simulink library "TestLib_BCM_Manager"  (Simulink 7.5)
settings: Solver=ode1  StartTime=0.0  StopTime=Inf  FixedStep=0.001  RelTol=1e-3
PostLoadFcn:
  | , if any(exist('dsrtsu_mdlpostloadfcn', 'file') == [2, 3, 6]), try dsrtsu_mdlpostloadfcn('Execute', bdroot); catch fprintf('Error in PostLoadFcn (dsrtsu_mdlpostloadfcn) for model "%s":\n %s\n', bdroot, lasterr); end, end,
undefined symbols (not defined in the file): cal, tloop
libraries: simulink x92, EC2_libraries x74
(part 1 of 2)
settings Model: DSRTSU_INTERNAL_RTI_VER=380  DSRTSU_INTERNAL_RTI_TYPE=rti1006  RTICANMMDATA=struct('GeneralSetupData',struct('modelroot',['C:\Users\EC2user\Documents\SVN__Controls\ecocar2_Controls\PTTR Alpha Branch\Libraries\CAN'],'generalsettings',struct('filesettings',struct('destfolder',struct('Name','RTICANMM_FILES','Check',1),'buildfolder',struct('Name','.','Check',1),'AbsDestfolder',struct('Name',['C:\Users\EC2user\Documents\SVN__Controls\ecocar2_Controls\PTTR Alpha Branch\Libraries\Diagnostics\Testing\RTICANMM_FILES']),'AbsBuildfolder',struct('Name',['C:\Users\EC2user\Documents\SVN__Controls\ecocar2_Controls\PTTR Alpha Branch\Libraries\CAN']))),'options',struct('addpaths',1,'rmpaths',1,'addtrcexclusion',logical(1),'cannavigator',struct('checkmonitoring',0,'serviceno','31','hostservicedefheader',struct('name','x','path','x')),'show_usrtrc',0,'use_usrtrc',0),'advanced',struct('options',[1 1 1 1 1 1 1 1 1 1 1 1 1 1 1 1 1 1 1 1 1 1 1 1 1 1 1 1 1 1 1 1 1 1 1 1 1 1 1 1 1 1 1 1 1 1 1 1 1 1 1 1 1 1 1 1 1 1 1 1 1 1 1 1 1 1 1 1 1 1 1 1 1 1 1 1 1 1 1 1 1 1 1 1 1 1 1 1 1 1 1 1 1 1 1 1 1 1 1 1]),'MPSetup',{{}},'modelname','DIAG_CAN_OUT','block','TestLib_BCM_Manager'))  Creator=idan  LastModifiedBy=Yuxia^_^

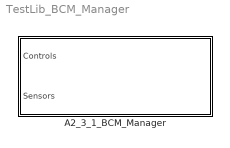
== system TestLib_BCM_Manager ==
  A2_3_1_BCM_Manager : Subsystem

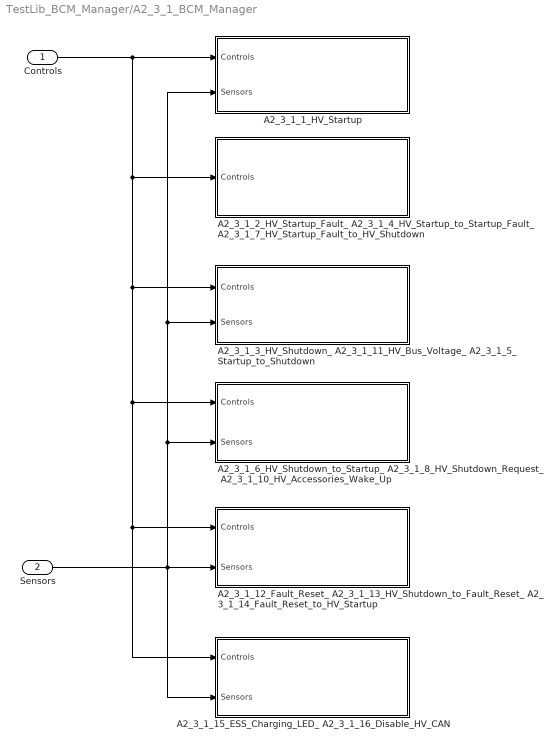
== system TestLib_BCM_Manager/A2_3_1_BCM_Manager ==
  Controls : Inport  OutDataType=fixdt(1, 16)  OutScaling=2^0
  Sensors : Inport  Port=2  OutDataType=fixdt(1, 16)  OutScaling=2^0
  A2_3_1_12_Fault_Reset_ A2_3_1_13_HV_Shutdown_to_Fault_Reset_ A2_3_1_14_Fault_Reset_to_HV_Startup : Subsystem
  A2_3_1_15_ESS_Charging_LED_ A2_3_1_16_Disable_HV_CAN : Subsystem
  A2_3_1_1_HV_Startup : Subsystem
  A2_3_1_2_HV_Startup_Fault_ A2_3_1_4_HV_Startup_to_Startup_Fault_ A2_3_1_7_HV_Startup_Fault_to_HV_Shutdown : Subsystem
  A2_3_1_3_HV_Shutdown_ A2_3_1_11_HV_Bus_Voltage_ A2_3_1_5_Startup_to_Shutdown : Subsystem
  A2_3_1_6_HV_Shutdown_to_Startup_ A2_3_1_8_HV_Shutdown_Request_ A2_3_1_10_HV_Accessories_Wake_Up : Subsystem
  wires:
  Controls/1 -> A2_3_1_15_ESS_Charging_LED_ A2_3_1_16_Disable_HV_CAN/1(Controls), A2_3_1_12_Fault_Reset_ A2_3_1_13_HV_Shutdown_to_Fault_Reset_ A2_3_1_14_Fault_Reset_to_HV_Startup/1(Controls), A2_3_1_6_HV_Shutdown_to_Startup_ A2_3_1_8_HV_Shutdown_Request_ A2_3_1_10_HV_Accessories_Wake_Up/1(Controls), A2_3_1_3_HV_Shutdown_ A2_3_1_11_HV_Bus_Voltage_ A2_3_1_5_Startup_to_Shutdown/1(Controls), A2_3_1_2_HV_Startup_Fault_ A2_3_1_4_HV_Startup_to_Startup_Fault_ A2_3_1_7_HV_Startup_Fault_to_HV_Shutdown/1(Controls), A2_3_1_1_HV_Startup/1(Controls)
  Sensors/1 -> A2_3_1_15_ESS_Charging_LED_ A2_3_1_16_Disable_HV_CAN/2(Sensors), A2_3_1_12_Fault_Reset_ A2_3_1_13_HV_Shutdown_to_Fault_Reset_ A2_3_1_14_Fault_Reset_to_HV_Startup/2(Sensors), A2_3_1_6_HV_Shutdown_to_Startup_ A2_3_1_8_HV_Shutdown_Request_ A2_3_1_10_HV_Accessories_Wake_Up/2(Sensors), A2_3_1_3_HV_Shutdown_ A2_3_1_11_HV_Bus_Voltage_ A2_3_1_5_Startup_to_Shutdown/2(Sensors), A2_3_1_1_HV_Startup/2(Sensors)

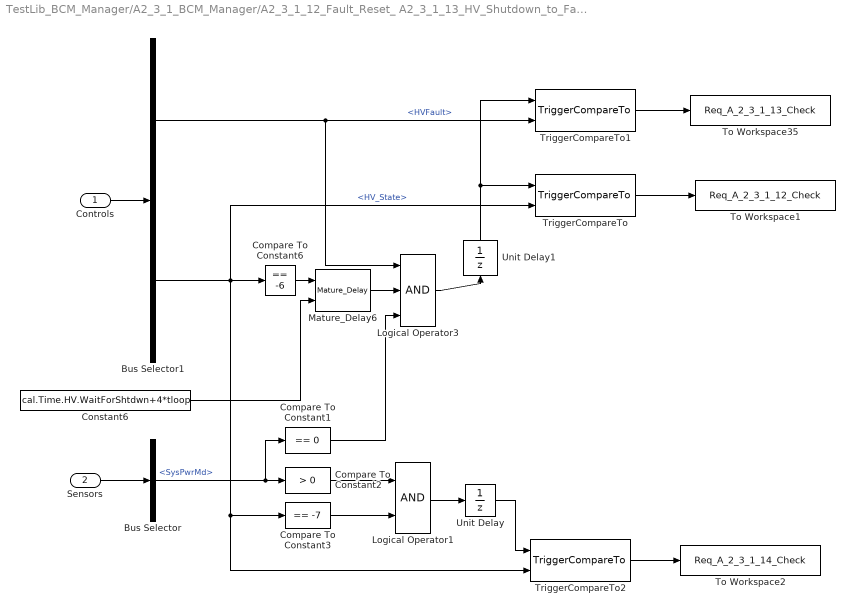
== system TestLib_BCM_Manager/A2_3_1_BCM_Manager/A2_3_1_12_Fault_Reset_ A2_3_1_13_HV_Shutdown_to_Fault_Reset_ A2_3_1_14_Fault_Reset_to_HV_Startup ==
  Controls : Inport  OutDataType=fixdt(1, 16)  OutScaling=2^0
  Sensors : Inport  Port=2  OutDataType=fixdt(1, 16)  OutScaling=2^0
  Bus Selector : BusSelector  OutputSignals=Sensors_CAN.BodyCM_HS_Tx.PPEI_Platform_General_Status.SysPwrMd
  Bus Selector1 : BusSelector  OutputSignals=Powertrain_SC_Controls.HV_Status.HVFault,Powertrain_SC_Controls.HV_Status.HV_State
  Compare To Constant1 : simulink/Logic and Bit Operations/Compare To Constant  SystemSampleTime=-1  relop===  const=0  LogicOutDataTypeMode=uint8
  Compare To Constant2 : simulink/Logic and Bit Operations/Compare To Constant  SystemSampleTime=-1  relop=>  const=0  LogicOutDataTypeMode=uint8
  Compare To Constant3 : simulink/Logic and Bit Operations/Compare To Constant  SystemSampleTime=-1  relop===  const=-7  LogicOutDataTypeMode=uint8
  Compare To Constant6 : simulink/Logic and Bit Operations/Compare To Constant  SystemSampleTime=-1  relop===  const=-6  LogicOutDataTypeMode=uint8
  Constant6 : Constant  Value=cal.Time.HV.WaitForShtdwn+4*tloop  VectorParams1D=off
  Logical Operator1 : Logic  AllPortsSameDT=off  OutDataTypeMode=boolean  OutDataTypeStr=boolean
  Logical Operator3 : Logic  Inputs=3  AllPortsSameDT=off  OutDataTypeMode=boolean  OutDataTypeStr=boolean
  Mature_Delay6 : EC2_libraries/Mature_Delay  SystemSampleTime=-1
  To Workspace1 : ToWorkspace  VariableName=Req_A_2_3_1_12_Check  SampleTime=-1  SaveFormat=Array
      settings: Decimation=WORKSPACE_DECIMATION
  To Workspace2 : ToWorkspace  VariableName=Req_A_2_3_1_14_Check  SampleTime=-1  SaveFormat=Array
      settings: Decimation=WORKSPACE_DECIMATION
  To Workspace35 : ToWorkspace  VariableName=Req_A_2_3_1_13_Check  SampleTime=-1  SaveFormat=Array
      settings: Decimation=WORKSPACE_DECIMATION
  TriggerCompareTo : EC2_libraries/TriggerCompareTo  SystemSampleTime=-1  exp_val=-7
  TriggerCompareTo1 : EC2_libraries/TriggerCompareTo  SystemSampleTime=-1  exp_val=0
  TriggerCompareTo2 : EC2_libraries/TriggerCompareTo  SystemSampleTime=-1  exp_val=-7
  Unit Delay : UnitDelay  SampleTime=-1
  Unit Delay1 : UnitDelay  SampleTime=-1
  wires:
  Unit Delay/1 -> TriggerCompareTo2/1
  Logical Operator1/1 -> Unit Delay/1
  Compare To Constant3/1 -> Logical Operator1/2
  Compare To Constant2/1 -> Logical Operator1/1
  TriggerCompareTo2/1 -> To Workspace2/1
  Logical Operator3/1 -> Unit Delay1/1
  TriggerCompareTo1/1 -> To Workspace35/1
  Bus Selector/1 -> Compare To Constant2/1, Compare To Constant1/1  "<SysPwrMd>"
  Bus Selector1/2 -> TriggerCompareTo/2, TriggerCompareTo2/2, Compare To Constant3/1, Compare To Constant6/1  "<HV_State>"
  Bus Selector1/1 -> TriggerCompareTo1/2, Logical Operator3/1  "<HVFault>"
  Controls/1 -> Bus Selector1/1
  Sensors/1 -> Bus Selector/1
  TriggerCompareTo/1 -> To Workspace1/1
  Unit Delay1/1 -> TriggerCompareTo1/1, TriggerCompareTo/1
  Compare To Constant1/1 -> Logical Operator3/3
  Constant6/1 -> Mature_Delay6/2
  Compare To Constant6/1 -> Mature_Delay6/1
  Mature_Delay6/1 -> Logical Operator3/2

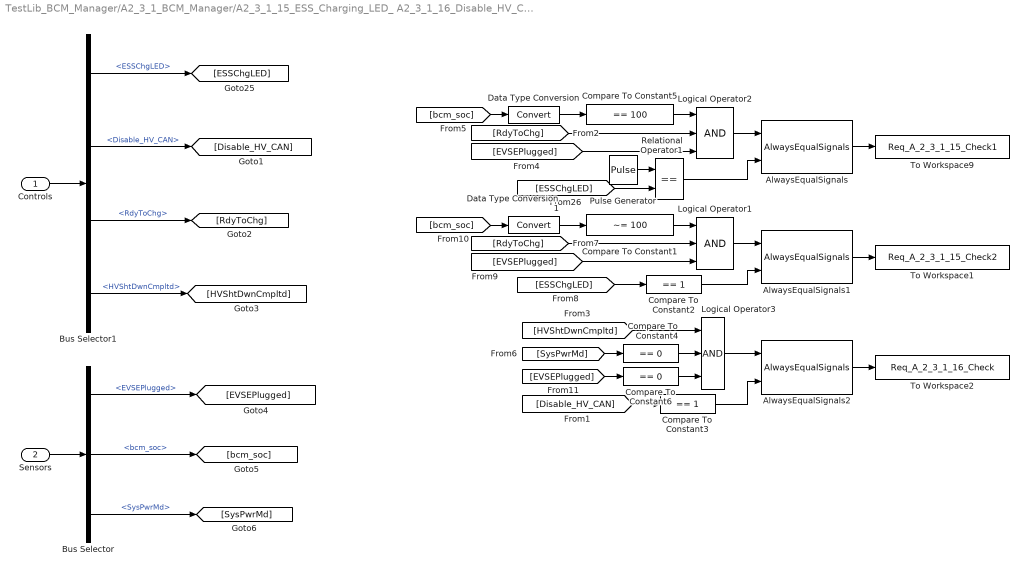
== system TestLib_BCM_Manager/A2_3_1_BCM_Manager/A2_3_1_15_ESS_Charging_LED_ A2_3_1_16_Disable_HV_CAN ==
  Controls : Inport  OutDataType=fixdt(1, 16)  OutScaling=2^0
  Sensors : Inport  Port=2  OutDataType=fixdt(1, 16)  OutScaling=2^0
  AlwaysEqualSignals : EC2_libraries/AlwaysEqualSignals  SystemSampleTime=-1
  AlwaysEqualSignals1 : EC2_libraries/AlwaysEqualSignals  SystemSampleTime=-1
  AlwaysEqualSignals2 : EC2_libraries/AlwaysEqualSignals  SystemSampleTime=-1
  Bus Selector : BusSelector  OutputSignals=Analog.EVSEPlugged,Sensors_CAN.BCM_HS_Tx.BCM_Status.bcm_soc,Sensors_CAN.BodyCM_HS_Tx.PPEI_Platform_General_Status.SysPwrMd
  Bus Selector1 : BusSelector  OutputSignals=Powertrain_SC_Controls.BCM_Control.ESSChgLED,Powertrain_SC_Controls.BCM_Control.Disable_HV_CAN,Powertrain_SC_Controls.HV_Status.RdyToChg,Powertrain_SC_Controls.HV_Status.HVShtDwnCmpltd
  Compare To Constant1 : simulink/Logic and Bit Operations/Compare To Constant  SystemSampleTime=-1  relop=~=  const=100  LogicOutDataTypeMode=boolean
  Compare To Constant2 : simulink/Logic and Bit Operations/Compare To Constant  SystemSampleTime=-1  relop===  const=1  LogicOutDataTypeMode=boolean
  Compare To Constant3 : simulink/Logic and Bit Operations/Compare To Constant  SystemSampleTime=-1  relop===  const=1  LogicOutDataTypeMode=boolean
  Compare To Constant4 : simulink/Logic and Bit Operations/Compare To Constant  SystemSampleTime=-1  relop===  const=0  LogicOutDataTypeMode=boolean
  Compare To Constant5 : simulink/Logic and Bit Operations/Compare To Constant  SystemSampleTime=-1  relop===  const=100  LogicOutDataTypeMode=boolean
  Compare To Constant6 : simulink/Logic and Bit Operations/Compare To Constant  SystemSampleTime=-1  relop===  const=0  LogicOutDataTypeMode=boolean
  Data Type Conversion : DataTypeConversion  OutDataType=fixdt(1, 16)  OutScaling=2^0
  Data Type Conversion1 : DataTypeConversion  OutDataType=fixdt(1, 16)  OutScaling=2^0
  Logical Operator1 : Logic  Inputs=3  AllPortsSameDT=off  OutDataTypeMode=boolean  LogicDataType=fixdt(0, 8)  OutDataTypeStr=boolean
  Logical Operator2 : Logic  Inputs=3  AllPortsSameDT=off  OutDataTypeMode=boolean  LogicDataType=fixdt(0, 8)  OutDataTypeStr=boolean
  Logical Operator3 : Logic  Inputs=3  AllPortsSameDT=off  OutDataTypeMode=boolean  LogicDataType=fixdt(0, 8)  OutDataTypeStr=boolean
  Pulse Generator : DiscretePulseGenerator  PulseType=Time based  Amplitude=1  Period=1  PulseWidth=50  PhaseDelay=0  SampleTime=1
  Relational Operator1 : RelationalOperator  Operator===  LogicOutDataTypeMode=boolean  LogicDataType=fixdt(0, 8)  OutDataTypeStr=boolean
  To Workspace1 : ToWorkspace  VariableName=Req_A_2_3_1_15_Check2  SampleTime=-1  SaveFormat=Array
      settings: Decimation=WORKSPACE_DECIMATION
  To Workspace2 : ToWorkspace  VariableName=Req_A_2_3_1_16_Check  SampleTime=-1  SaveFormat=Array
      settings: Decimation=WORKSPACE_DECIMATION
  To Workspace9 : ToWorkspace  VariableName=Req_A_2_3_1_15_Check1  SampleTime=-1  SaveFormat=Array
      settings: Decimation=WORKSPACE_DECIMATION
  wires:
  Compare To Constant6/1 -> Logical Operator3/3
  Compare To Constant4/1 -> Logical Operator3/2
  [Disable_HV_CAN] -> Compare To Constant3/1
  Logical Operator3/1 -> AlwaysEqualSignals2/1
  Compare To Constant3/1 -> AlwaysEqualSignals2/2
  [SysPwrMd] -> Compare To Constant4/1
  [EVSEPlugged] -> Compare To Constant6/1
  [HVShtDwnCmpltd] -> Logical Operator3/1
  AlwaysEqualSignals2/1 -> To Workspace2/1
  [ESSChgLED] -> Compare To Constant2/1
  Logical Operator1/1 -> AlwaysEqualSignals1/1
  Compare To Constant2/1 -> AlwaysEqualSignals1/2
  [bcm_soc] -> Data Type Conversion1/1
  [RdyToChg] -> Logical Operator1/2
  [EVSEPlugged] -> Logical Operator1/3
  Data Type Conversion1/1 -> Compare To Constant1/1
  Compare To Constant1/1 -> Logical Operator1/1
  AlwaysEqualSignals1/1 -> To Workspace1/1
  Logical Operator2/1 -> AlwaysEqualSignals/1
  Relational Operator1/1 -> AlwaysEqualSignals/2
  [ESSChgLED] -> Relational Operator1/2
  [bcm_soc] -> Data Type Conversion/1
  [RdyToChg] -> Logical Operator2/2
  [EVSEPlugged] -> Logical Operator2/3
  Pulse Generator/1 -> Relational Operator1/1
  Data Type Conversion/1 -> Compare To Constant5/1
  Compare To Constant5/1 -> Logical Operator2/1
  AlwaysEqualSignals/1 -> To Workspace9/1
  Bus Selector/3 -> [SysPwrMd]  "<SysPwrMd>"
  Bus Selector/2 -> [bcm_soc]  "<bcm_soc>"
  Bus Selector/1 -> [EVSEPlugged]  "<EVSEPlugged>"
  Bus Selector1/4 -> [HVShtDwnCmpltd]  "<HVShtDwnCmpltd>"
  Bus Selector1/3 -> [RdyToChg]  "<RdyToChg>"
  Bus Selector1/2 -> [Disable_HV_CAN]  "<Disable_HV_CAN>"
  Bus Selector1/1 -> [ESSChgLED]  "<ESSChgLED>"
  Sensors/1 -> Bus Selector/1
  Controls/1 -> Bus Selector1/1

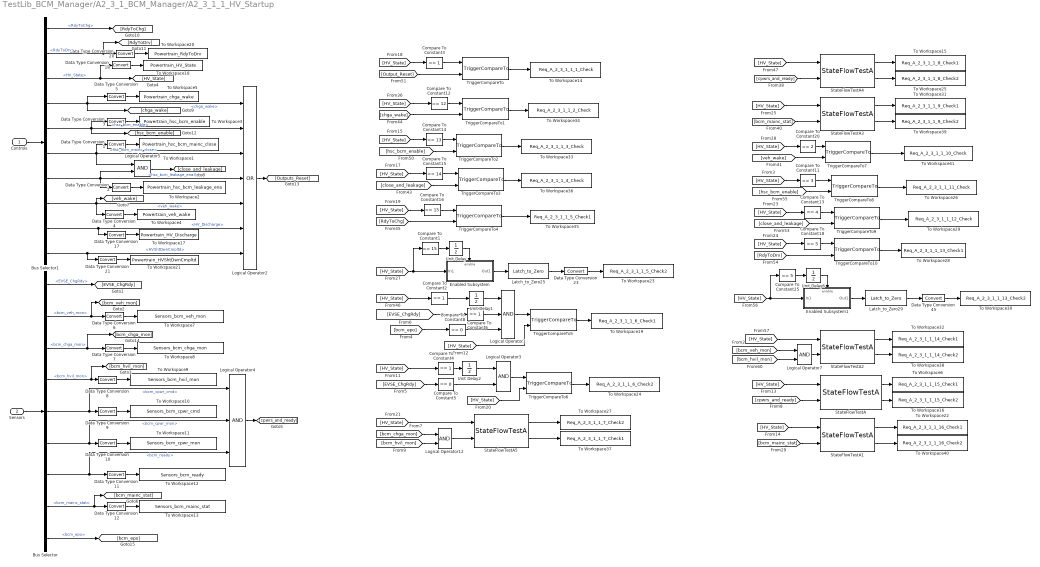
== system TestLib_BCM_Manager/A2_3_1_BCM_Manager/A2_3_1_1_HV_Startup ==
  Controls : Inport  OutDataType=fixdt(1, 16)  OutScaling=2^0
  Sensors : Inport  Port=2  OutDataType=fixdt(1, 16)  OutScaling=2^0
  Bus Selector : BusSelector  OutputSignals=Analog.EVSE_ChgRdy,Sensors_CAN.BCM_HS_Tx.BCM_Data1.bcm_veh_mon,Sensors_CAN.BCM_HS_Tx.BCM_Data1.bcm_chga_mon,Sensors_CAN.BCM_HS_Tx.BCM_Status.bcm_hvil_mon,Sensors_CAN.BCM_HS_Tx.BCM_Status.bcm_cpwr_cmd,Sensors_CAN.BCM_HS_Tx.BCM_Status.bcm_cpwr_mon,Sensors_CAN.BCM_HS_Tx.BCM_Status.bcm_ready,Sensors_CAN.BCM_HS_Tx.BCM_Status.bcm_mainc_stat,Sensors_CAN.BCM_HS_Tx.BCM_Status.bcm_epo
  Bus Selector1 : BusSelector  OutputSignals=Powertrain_SC_Controls.HV_Status.RdyToChg,Powertrain_SC_Controls.HV_Status.RdyToDrv,Powertrain_SC_Controls.HV_Status.HV_State,Powertrain_SC_Controls.BCM_Control.chga_wake,Powertrain_SC_Controls.BCM_Control.hsc_bcm_enable,Powertrain_SC_Controls.BCM_Control.hsc_bcm_mainc_close,Powertrain_SC_Controls.BCM_Control.hsc_bcm_leakage_ena,Powertrain_SC_Controls.BCM_Control.veh_wake,Powertrain_SC_Controls.HV_Status.HV_Discharge,Powertrain_SC_Controls.HV_Status.HVShtDwnCmpltd
  Compare To Constant1 : simulink/Logic and Bit Operations/Compare To Constant  SystemSampleTime=-1  relop===  const=15  LogicOutDataTypeMode=uint8
  Compare To Constant11 : simulink/Logic and Bit Operations/Compare To Constant  SystemSampleTime=-1  relop===  const=3  LogicOutDataTypeMode=uint8
  Compare To Constant12 : simulink/Logic and Bit Operations/Compare To Constant  SystemSampleTime=-1  relop===  const=12  LogicOutDataTypeMode=uint8
  Compare To Constant13 : simulink/Logic and Bit Operations/Compare To Constant  SystemSampleTime=-1  relop===  const=4  LogicOutDataTypeMode=uint8
  Compare To Constant14 : simulink/Logic and Bit Operations/Compare To Constant  SystemSampleTime=-1  relop===  const=13  LogicOutDataTypeMode=uint8
  Compare To Constant15 : simulink/Logic and Bit Operations/Compare To Constant  SystemSampleTime=-1  relop===  const=14  LogicOutDataTypeMode=uint8
  Compare To Constant16 : simulink/Logic and Bit Operations/Compare To Constant  SystemSampleTime=-1  relop===  const=15  LogicOutDataTypeMode=uint8
  Compare To Constant18 : simulink/Logic and Bit Operations/Compare To Constant  SystemSampleTime=-1  relop===  const=5  LogicOutDataTypeMode=uint8
  Compare To Constant{2..4,6} (4 alike) : simulink/Logic and Bit Operations/Compare To Constant  SystemSampleTime=-1  relop===  const=1  LogicOutDataTypeMode=uint8
  Compare To Constant20 : simulink/Logic and Bit Operations/Compare To Constant  SystemSampleTime=-1  relop===  const=2  LogicOutDataTypeMode=uint8
  Compare To Constant25 : simulink/Logic and Bit Operations/Compare To Constant  SystemSampleTime=-1  relop===  const=5  LogicOutDataTypeMode=uint8
  Compare To Constant5 : simulink/Logic and Bit Operations/Compare To Constant  SystemSampleTime=-1  relop===  const=0  LogicOutDataTypeMode=uint8
  Compare To Constant8 : simulink/Logic and Bit Operations/Compare To Constant  SystemSampleTime=-1  relop===  const=0  LogicOutDataTypeMode=uint8
  Data Type Conversion{1..12,17..18,20..21,23,45} (18 alike) : DataTypeConversion  OutDataType=fixdt(1, 16)  OutScaling=2^0
  Enabled Subsystem : Subsystem  TreatAsAtomicUnit=on
  Enabled Subsystem1 : Subsystem  TreatAsAtomicUnit=on
  Latch_to_Zero25 : EC2_libraries/Latch_to_Zero  SystemSampleTime=-1
  Latch_to_Zero29 : EC2_libraries/Latch_to_Zero  SystemSampleTime=-1
  Logical Operator1 : Logic  Inputs=3  AllPortsSameDT=off  OutDataTypeMode=boolean  OutDataTypeStr=boolean
  Logical Operator{3,5,7,12} (4 alike) : Logic  AllPortsSameDT=off  OutDataTypeMode=boolean  OutDataTypeStr=boolean
  Logical Operator2 : Logic  Operator=OR  Inputs=7  AllPortsSameDT=off  OutDataTypeMode=boolean  OutDataTypeStr=boolean
  Logical Operator4 : Logic  Inputs=3  AllPortsSameDT=off  OutDataTypeMode=boolean  OutDataTypeStr=boolean
  StateFlowTestA : EC2_libraries/StateFlowTestA  SystemSampleTime=-1  State=3
  StateFlowTestA1 : EC2_libraries/StateFlowTestA  SystemSampleTime=-1  State=4
  StateFlowTestA2 : EC2_libraries/StateFlowTestA  SystemSampleTime=-1  State=2
  StateFlowTestA3 : EC2_libraries/StateFlowTestA  SystemSampleTime=-1  State=14
  StateFlowTestA4 : EC2_libraries/StateFlowTestA  SystemSampleTime=-1  State=13
  StateFlowTestA5 : EC2_libraries/StateFlowTestA  SystemSampleTime=-1  State=12
  To Workspace1 : ToWorkspace  VariableName=Powertrain_hsc_bcm_mainc_close  SampleTime=-1  SaveFormat=Array
      settings: Decimation=WORKSPACE_DECIMATION
  To Workspace10 : ToWorkspace  VariableName=Sensors_bcm_cpwr_cmd  SampleTime=-1  SaveFormat=Array
      settings: Decimation=WORKSPACE_DECIMATION
  To Workspace11 : ToWorkspace  VariableName=Sensors_bcm_cpwr_mon  SampleTime=-1  SaveFormat=Array
      settings: Decimation=WORKSPACE_DECIMATION
  To Workspace12 : ToWorkspace  VariableName=Sensors_bcm_ready  SampleTime=-1  SaveFormat=Array
      settings: Decimation=WORKSPACE_DECIMATION
  To Workspace13 : ToWorkspace  VariableName=Sensors_bcm_mainc_stat  SampleTime=-1  SaveFormat=Array
      settings: Decimation=WORKSPACE_DECIMATION
  To Workspace14 : ToWorkspace  VariableName=Req_A_2_3_1_1_1_Check  SampleTime=-1  SaveFormat=Array
      settings: Decimation=WORKSPACE_DECIMATION
  To Workspace15 : ToWorkspace  VariableName=Req_A_2_3_1_1_8_Check1  SampleTime=-1  SaveFormat=Array
      settings: Decimation=WORKSPACE_DECIMATION
  To Workspace16 : ToWorkspace  VariableName=Req_A_2_3_1_1_15_Check2  SampleTime=-1  SaveFormat=Array
      settings: Decimation=WORKSPACE_DECIMATION
  To Workspace17 : ToWorkspace  VariableName=Powertrain_HV_Discharge  SampleTime=-1  SaveFormat=Array
      settings: Decimation=WORKSPACE_DECIMATION
  To Workspace18 : ToWorkspace  VariableName=Powertrain_HV_State  SampleTime=-1  SaveFormat=Array
      settings: Decimation=WORKSPACE_DECIMATION
  To Workspace19 : ToWorkspace  VariableName=Req_A_2_3_1_1_6_Check1  SampleTime=-1  SaveFormat=Array
      settings: Decimation=WORKSPACE_DECIMATION
  To Workspace2 : ToWorkspace  VariableName=Powertrain_hsc_bcm_leakage_ena  SampleTime=-1  SaveFormat=Array
      settings: Decimation=WORKSPACE_DECIMATION
  To Workspace20 : ToWorkspace  VariableName=Powertrain_RdyToDrv  SampleTime=-1  SaveFormat=Array
      settings: Decimation=WORKSPACE_DECIMATION
  To Workspace21 : ToWorkspace  VariableName=Powertrain_HVShtDwnCmpltd  SampleTime=-1  SaveFormat=Array
      settings: Decimation=WORKSPACE_DECIMATION
  To Workspace22 : ToWorkspace  VariableName=Req_A_2_3_1_1_16_Check1  SampleTime=-1  SaveFormat=Array
      settings: Decimation=WORKSPACE_DECIMATION
  To Workspace23 : ToWorkspace  VariableName=Req_A_2_3_1_1_5_Check2  SampleTime=-1  SaveFormat=Array
      settings: Decimation=WORKSPACE_DECIMATION
  To Workspace24 : ToWorkspace  VariableName=Req_A_2_3_1_1_6_Check2  SampleTime=-1  SaveFormat=Array
      settings: Decimation=WORKSPACE_DECIMATION
  To Workspace25 : ToWorkspace  VariableName=Req_A_2_3_1_1_8_Check2  SampleTime=-1  SaveFormat=Array
      settings: Decimation=WORKSPACE_DECIMATION
  To Workspace26 : ToWorkspace  VariableName=Req_A_2_3_1_1_11_Check  SampleTime=-1  SaveFormat=Array
      settings: Decimation=WORKSPACE_DECIMATION
  To Workspace27 : ToWorkspace  VariableName=Req_A_2_3_1_1_7_Check2  SampleTime=-1  SaveFormat=Array
      settings: Decimation=WORKSPACE_DECIMATION
  To Workspace28 : ToWorkspace  VariableName=Req_A_2_3_1_1_13_Check1  SampleTime=-1  SaveFormat=Array
      settings: Decimation=WORKSPACE_DECIMATION
  To Workspace29 : ToWorkspace  VariableName=Req_A_2_3_1_1_12_Check  SampleTime=-1  SaveFormat=Array
      settings: Decimation=WORKSPACE_DECIMATION
  To Workspace3 : ToWorkspace  VariableName=Powertrain_hsc_bcm_enable  SampleTime=-1  SaveFormat=Array
      settings: Decimation=WORKSPACE_DECIMATION
  To Workspace30 : ToWorkspace  VariableName=Req_A_2_3_1_1_13_Check2  SampleTime=-1  SaveFormat=Array
      settings: Decimation=WORKSPACE_DECIMATION
  To Workspace31 : ToWorkspace  VariableName=Req_A_2_3_1_1_9_Check1  SampleTime=-1  SaveFormat=Array
      settings: Decimation=WORKSPACE_DECIMATION
  To Workspace32 : ToWorkspace  VariableName=Req_A_2_3_1_1_14_Check1  SampleTime=-1  SaveFormat=Array
      settings: Decimation=WORKSPACE_DECIMATION
  To Workspace33 : ToWorkspace  VariableName=Req_A_2_3_1_1_3_Check  SampleTime=-1  SaveFormat=Array
      settings: Decimation=WORKSPACE_DECIMATION
  To Workspace34 : ToWorkspace  VariableName=Req_A_2_3_1_1_2_Check  SampleTime=-1  SaveFormat=Array
      settings: Decimation=WORKSPACE_DECIMATION
  To Workspace35 : ToWorkspace  VariableName=Req_A_2_3_1_1_5_Check1  SampleTime=-1  SaveFormat=Array
      settings: Decimation=WORKSPACE_DECIMATION
  To Workspace36 : ToWorkspace  VariableName=Req_A_2_3_1_1_4_Check  SampleTime=-1  SaveFormat=Array
      settings: Decimation=WORKSPACE_DECIMATION
  To Workspace37 : ToWorkspace  VariableName=Req_A_2_3_1_1_7_Check1  SampleTime=-1  SaveFormat=Array
      settings: Decimation=WORKSPACE_DECIMATION
  To Workspace38 : ToWorkspace  VariableName=Req_A_2_3_1_1_14_Check2  SampleTime=-1  SaveFormat=Array
      settings: Decimation=WORKSPACE_DECIMATION
  To Workspace39 : ToWorkspace  VariableName=Req_A_2_3_1_1_9_Check2  SampleTime=-1  SaveFormat=Array
      settings: Decimation=WORKSPACE_DECIMATION
  To Workspace4 : ToWorkspace  VariableName=Powertrain_veh_wake  SampleTime=-1  SaveFormat=Array
      settings: Decimation=WORKSPACE_DECIMATION
  To Workspace40 : ToWorkspace  VariableName=Req_A_2_3_1_1_16_Check2  SampleTime=-1  SaveFormat=Array
      settings: Decimation=WORKSPACE_DECIMATION
  To Workspace41 : ToWorkspace  VariableName=Req_A_2_3_1_1_10_Check  SampleTime=-1  SaveFormat=Array
      settings: Decimation=WORKSPACE_DECIMATION
  To Workspace5 : ToWorkspace  VariableName=Powertrain_chga_wake  SampleTime=-1  SaveFormat=Array
      settings: Decimation=WORKSPACE_DECIMATION
  To Workspace6 : ToWorkspace  VariableName=Req_A_2_3_1_1_15_Check1  SampleTime=-1  SaveFormat=Array
      settings: Decimation=WORKSPACE_DECIMATION
  To Workspace7 : ToWorkspace  VariableName=Sensors_bcm_veh_mon  SampleTime=-1  SaveFormat=Array
      settings: Decimation=WORKSPACE_DECIMATION
  To Workspace8 : ToWorkspace  VariableName=Sensors_bcm_chga_mon  SampleTime=-1  SaveFormat=Array
      settings: Decimation=WORKSPACE_DECIMATION
  To Workspace9 : ToWorkspace  VariableName=Sensors_bcm_hvil_mon  SampleTime=-1  SaveFormat=Array
      settings: Decimation=WORKSPACE_DECIMATION
  TriggerCompareTo : EC2_libraries/TriggerCompareTo  SystemSampleTime=-1  exp_val=0
  TriggerCompareTo{1..4,7..10} (8 alike) : EC2_libraries/TriggerCompareTo  SystemSampleTime=-1  exp_val=1
  TriggerCompareTo5 : EC2_libraries/TriggerCompareTo  SystemSampleTime=-1  exp_val=12
  TriggerCompareTo6 : EC2_libraries/TriggerCompareTo  SystemSampleTime=-1  exp_val=2
  Unit Delay{,1..2,6} (4 alike) : UnitDelay  SampleTime=-1
  wires:
  [HV_State] -> StateFlowTestA5/1
  Logical Operator12/1 -> StateFlowTestA5/2
  StateFlowTestA3/2 -> To Workspace39/1
  [bcm_mainc_stat] -> StateFlowTestA3/2
  [HV_State] -> StateFlowTestA3/1
  [cpwrs_and_ready] -> StateFlowTestA4/2
  [HV_State] -> StateFlowTestA4/1
  [HV_State] -> StateFlowTestA2/1
  Logical Operator7/1 -> StateFlowTestA2/2
  StateFlowTestA1/2 -> To Workspace40/1
  [bcm_mainc_stat] -> StateFlowTestA1/2
  [HV_State] -> StateFlowTestA1/1
  [HV_State] -> StateFlowTestA/1
  [cpwrs_and_ready] -> StateFlowTestA/2
  Compare To Constant13/1 -> TriggerCompareTo9/1
  TriggerCompareTo7/1 -> To Workspace41/1
  StateFlowTestA3/1 -> To Workspace31/1
  StateFlowTestA1/1 -> To Workspace22/1
  StateFlowTestA/2 -> To Workspace16/1
  StateFlowTestA/1 -> To Workspace6/1
  StateFlowTestA2/2 -> To Workspace38/1
  [bcm_hvil_mon] -> Logical Operator7/2
  [bcm_veh_mon] -> Logical Operator7/1
  StateFlowTestA2/1 -> To Workspace32/1
  Compare To Constant25/1 -> Unit Delay6/1
  Unit Delay6/1 -> Enabled Subsystem1/Enable
  Data Type Conversion45/1 -> To Workspace30/1
  [HV_State] -> Compare To Constant25/1, Enabled Subsystem1/1(In1)
  Latch_to_Zero29/1 -> Data Type Conversion45/1
  Enabled Subsystem1/1(Out1) -> Latch_to_Zero29/1
  [hsc_bcm_enable] -> TriggerCompareTo8/2
  [close_and_leakage] -> TriggerCompareTo9/2
  [HV_State] -> Compare To Constant13/1
  Compare To Constant11/1 -> TriggerCompareTo8/1
  [RdyToDrv] -> TriggerCompareTo10/2
  [HV_State] -> Compare To Constant11/1
  [HV_State] -> Compare To Constant18/1
  Compare To Constant18/1 -> TriggerCompareTo10/1
  TriggerCompareTo10/1 -> To Workspace28/1
  TriggerCompareTo9/1 -> To Workspace29/1
  TriggerCompareTo8/1 -> To Workspace26/1
  StateFlowTestA4/2 -> To Workspace25/1
  StateFlowTestA4/1 -> To Workspace15/1
  [bcm_hvil_mon] -> Logical Operator12/2
  [bcm_chga_mon] -> Logical Operator12/1
  Unit Delay1/1 -> Logical Operator1/1
  Compare To Constant2/1 -> Unit Delay1/1
  Logical Operator3/1 -> TriggerCompareTo6/1
  Compare To Constant5/1 -> Logical Operator3/2
  Compare To Constant4/1 -> Unit Delay2/1
  Unit Delay2/1 -> Logical Operator3/1
  [HV_State] -> Compare To Constant4/1
  [EVSE_ChgRdy] -> Compare To Constant5/1
  Logical Operator1/1 -> TriggerCompareTo5/1
  Compare To Constant6/1 -> Logical Operator1/2
  [HV_State] -> Compare To Constant2/1
  Compare To Constant1/1 -> Unit Delay/1
  Unit Delay/1 -> Enabled Subsystem/Enable
  [hsc_bcm_enable] -> TriggerCompareTo2/2
  [close_and_leakage] -> TriggerCompareTo3/2
  [HV_State] -> Compare To Constant15/1
  Compare To Constant15/1 -> TriggerCompareTo3/1
  Compare To Constant14/1 -> TriggerCompareTo2/1
  Data Type Conversion23/1 -> To Workspace23/1
  Bus Selector1/4 -> Data Type Conversion5/1, Logical Operator2/1, [chga_wake]  "<chga_wake>"
  Bus Selector1/5 -> Data Type Conversion3/1, Logical Operator2/2, [hsc_bcm_enable]  "<hsc_bcm_enable>"
  Bus Selector1/6 -> Data Type Conversion1/1, Logical Operator2/3, Logical Operator5/1  "<hsc_bcm_mainc_close>"
  Bus Selector1/7 -> Logical Operator5/2, Logical Operator2/4, Data Type Conversion2/1  "<hsc_bcm_leakage_ena>"
  Bus Selector1/8 -> Data Type Conversion4/1, Logical Operator2/5, [veh_wake]  "<veh_wake>"
  [Output_Reset] -> TriggerCompareTo/2
  Logical Operator2/1 -> [Outputs_Reset]
  Bus Selector1/1 -> [RdyToChg]  "<RdyToChg>"
  [RdyToChg] -> TriggerCompareTo4/2
  [chga_wake] -> TriggerCompareTo1/2
  Logical Operator5/1 -> [close_and_leakage]
  [veh_wake] -> TriggerCompareTo7/2
  Logical Operator4/1 -> [cpwrs_and_ready]
  [HV_State] -> Compare To Constant3/1
  [HV_State] -> Compare To Constant14/1
  [HV_State] -> Compare To Constant12/1
  [HV_State] -> Compare To Constant16/1
  [HV_State] -> TriggerCompareTo5/2
  [HV_State] -> TriggerCompareTo6/2
  [HV_State] -> Compare To Constant1/1, Enabled Subsystem/1(In1)
  [HV_State] -> Compare To Constant20/1
  Bus Selector/1 -> [EVSE_ChgRdy]  "<EVSE_ChgRdy>"
  [EVSE_ChgRdy] -> Compare To Constant6/1
  Compare To Constant12/1 -> TriggerCompareTo1/1
  TriggerCompareTo/1 -> To Workspace14/1
  Compare To Constant3/1 -> TriggerCompareTo/1
  Compare To Constant20/1 -> TriggerCompareTo7/1
  Compare To Constant16/1 -> TriggerCompareTo4/1
  TriggerCompareTo4/1 -> To Workspace35/1
  TriggerCompareTo3/1 -> To Workspace36/1
  TriggerCompareTo2/1 -> To Workspace33/1
  TriggerCompareTo1/1 -> To Workspace34/1
  StateFlowTestA5/2 -> To Workspace37/1
  StateFlowTestA5/1 -> To Workspace27/1
  TriggerCompareTo6/1 -> To Workspace24/1
  TriggerCompareTo5/1 -> To Workspace19/1
  Bus Selector/5 -> Logical Operator4/1, Data Type Conversion9/1  "<bcm_cpwr_cmd>"
  Bus Selector/4 -> [bcm_hvil_mon], Data Type Conversion8/1  "<bcm_hvil_mon>"
  Bus Selector/3 -> [bcm_chga_mon], Data Type Conversion7/1  "<bcm_chga_mon>"
  Bus Selector/2 -> [bcm_veh_mon], Data Type Conversion6/1  "<bcm_veh_mon>"
  Bus Selector/6 -> Logical Operator4/2, Data Type Conversion10/1  "<bcm_cpwr_mon>"
  Bus Selector/7 -> Logical Operator4/3, Data Type Conversion11/1  "<bcm_ready>"
  Bus Selector/8 -> [bcm_mainc_stat], Data Type Conversion12/1  "<bcm_mainc_stat>"
  Data Type Conversion12/1 -> To Workspace13/1
  Data Type Conversion11/1 -> To Workspace12/1
  Data Type Conversion10/1 -> To Workspace11/1
  Data Type Conversion9/1 -> To Workspace10/1
  Data Type Conversion8/1 -> To Workspace9/1
  Data Type Conversion7/1 -> To Workspace8/1
  Data Type Conversion6/1 -> To Workspace7/1
  Bus Selector1/2 -> [RdyToDrv], Data Type Conversion20/1  "<RdyToDrv>"
  Data Type Conversion18/1 -> To Workspace18/1
  Bus Selector1/10 -> Data Type Conversion21/1, Logical Operator2/7  "<HVShtDwnCmpltd>"
  Bus Selector1/9 -> Data Type Conversion17/1, Logical Operator2/6  "<HV_Discharge>"
  Bus Selector1/3 -> [HV_State], Data Type Conversion18/1  "<HV_State>"
  Data Type Conversion20/1 -> To Workspace20/1
  Data Type Conversion21/1 -> To Workspace21/1
  Data Type Conversion17/1 -> To Workspace17/1
  Data Type Conversion5/1 -> To Workspace5/1
  Data Type Conversion4/1 -> To Workspace4/1
  Data Type Conversion2/1 -> To Workspace2/1
  Data Type Conversion1/1 -> To Workspace1/1
  Data Type Conversion3/1 -> To Workspace3/1
  Controls/1 -> Bus Selector1/1
  Sensors/1 -> Bus Selector/1
  Latch_to_Zero25/1 -> Data Type Conversion23/1
  Enabled Subsystem/1(Out1) -> Latch_to_Zero25/1
  Bus Selector/9 -> [bcm_epo]  "<bcm_epo>"
  [bcm_epo] -> Compare To Constant8/1
  Compare To Constant8/1 -> Logical Operator1/3

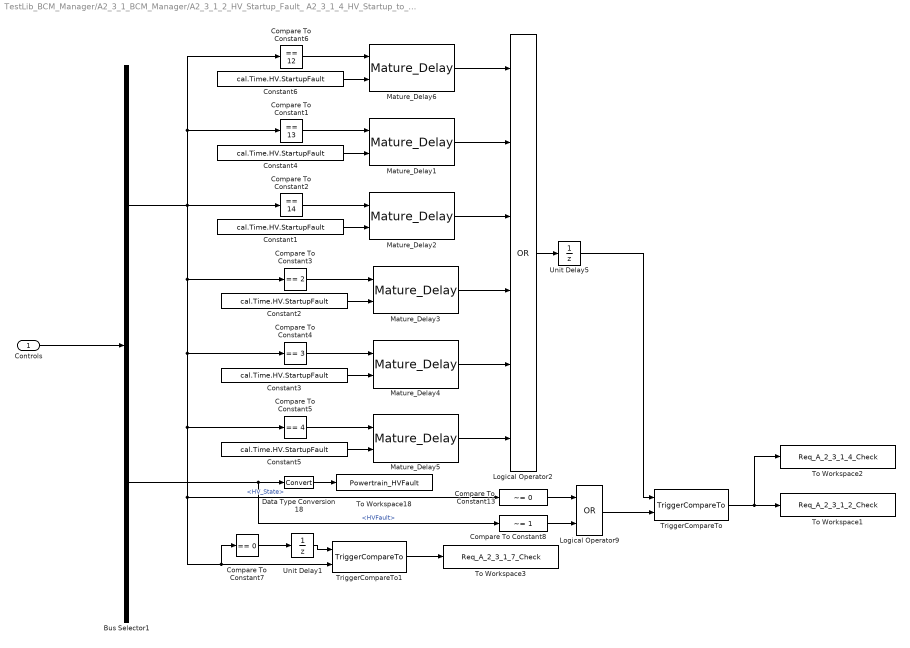
== system TestLib_BCM_Manager/A2_3_1_BCM_Manager/A2_3_1_2_HV_Startup_Fault_ A2_3_1_4_HV_Startup_to_Startup_Fault_ A2_3_1_7_HV_Startup_Fault_to_HV_Shutdown ==
  Controls : Inport  OutDataType=fixdt(1, 16)  OutScaling=2^0
  Bus Selector1 : BusSelector  OutputSignals=Powertrain_SC_Controls.HV_Status.HV_State,Powertrain_SC_Controls.HV_Status.HVFault
  Compare To Constant1 : simulink/Logic and Bit Operations/Compare To Constant  SystemSampleTime=-1  relop===  const=13  LogicOutDataTypeMode=uint8
  Compare To Constant13 : simulink/Logic and Bit Operations/Compare To Constant  SystemSampleTime=-1  relop=~=  const=0  LogicOutDataTypeMode=boolean
  Compare To Constant2 : simulink/Logic and Bit Operations/Compare To Constant  SystemSampleTime=-1  relop===  const=14  LogicOutDataTypeMode=uint8
  Compare To Constant3 : simulink/Logic and Bit Operations/Compare To Constant  SystemSampleTime=-1  relop===  const=2  LogicOutDataTypeMode=uint8
  Compare To Constant4 : simulink/Logic and Bit Operations/Compare To Constant  SystemSampleTime=-1  relop===  const=3  LogicOutDataTypeMode=uint8
  Compare To Constant5 : simulink/Logic and Bit Operations/Compare To Constant  SystemSampleTime=-1  relop===  const=4  LogicOutDataTypeMode=uint8
  Compare To Constant6 : simulink/Logic and Bit Operations/Compare To Constant  SystemSampleTime=-1  relop===  const=12  LogicOutDataTypeMode=uint8
  Compare To Constant7 : simulink/Logic and Bit Operations/Compare To Constant  SystemSampleTime=-1  relop===  const=0  LogicOutDataTypeMode=uint8
  Compare To Constant8 : simulink/Logic and Bit Operations/Compare To Constant  SystemSampleTime=-1  relop=~=  const=1  LogicOutDataTypeMode=boolean
  Constant{1..6} (6 alike) : Constant  Value=cal.Time.HV.StartupFault  VectorParams1D=off
  Data Type Conversion18 : DataTypeConversion  OutDataType=fixdt(1, 16)  OutScaling=2^0
  Logical Operator2 : Logic  Operator=OR  Inputs=6  AllPortsSameDT=off  OutDataTypeMode=boolean  OutDataTypeStr=boolean
  Logical Operator9 : Logic  Operator=OR  AllPortsSameDT=off  OutDataTypeMode=boolean  OutDataTypeStr=boolean
  Mature_Delay{1..6} (6 alike) : EC2_libraries/Mature_Delay  SystemSampleTime=-1
  To Workspace1 : ToWorkspace  VariableName=Req_A_2_3_1_2_Check  SampleTime=-1  SaveFormat=Array
      settings: Decimation=WORKSPACE_DECIMATION
  To Workspace18 : ToWorkspace  VariableName=Powertrain_HVFault  SampleTime=-1  SaveFormat=Array
      settings: Decimation=WORKSPACE_DECIMATION
  To Workspace2 : ToWorkspace  VariableName=Req_A_2_3_1_4_Check  SampleTime=-1  SaveFormat=Array
      settings: Decimation=WORKSPACE_DECIMATION
  To Workspace3 : ToWorkspace  VariableName=Req_A_2_3_1_7_Check  SampleTime=-1  SaveFormat=Array
      settings: Decimation=WORKSPACE_DECIMATION
  TriggerCompareTo : EC2_libraries/TriggerCompareTo  SystemSampleTime=-1  exp_val=0
  TriggerCompareTo1 : EC2_libraries/TriggerCompareTo  SystemSampleTime=-1  exp_val=-1
  Unit Delay1 : UnitDelay  SampleTime=-1
  Unit Delay5 : UnitDelay  SampleTime=-1
  wires:
  Logical Operator9/1 -> TriggerCompareTo/2
  Compare To Constant13/1 -> Logical Operator9/1
  Compare To Constant8/1 -> Logical Operator9/2
  TriggerCompareTo1/1 -> To Workspace3/1
  Logical Operator2/1 -> Unit Delay5/1
  TriggerCompareTo/1 -> To Workspace2/1, To Workspace1/1
  Constant6/1 -> Mature_Delay6/2
  Compare To Constant6/1 -> Mature_Delay6/1
  Mature_Delay6/1 -> Logical Operator2/1
  Constant5/1 -> Mature_Delay5/2
  Compare To Constant5/1 -> Mature_Delay5/1
  Mature_Delay5/1 -> Logical Operator2/6
  Constant3/1 -> Mature_Delay4/2
  Compare To Constant4/1 -> Mature_Delay4/1
  Mature_Delay4/1 -> Logical Operator2/5
  Constant2/1 -> Mature_Delay3/2
  Compare To Constant3/1 -> Mature_Delay3/1
  Mature_Delay3/1 -> Logical Operator2/4
  Constant1/1 -> Mature_Delay2/2
  Compare To Constant2/1 -> Mature_Delay2/1
  Mature_Delay2/1 -> Logical Operator2/3
  Constant4/1 -> Mature_Delay1/2
  Compare To Constant1/1 -> Mature_Delay1/1
  Mature_Delay1/1 -> Logical Operator2/2
  Data Type Conversion18/1 -> To Workspace18/1
  Bus Selector1/2 -> Compare To Constant8/1, Data Type Conversion18/1  "<HVFault>"
  Bus Selector1/1 -> Compare To Constant13/1, TriggerCompareTo1/2, Compare To Constant7/1, Compare To Constant5/1, Compare To Constant4/1, Compare To Constant3/1, Compare To Constant6/1, Compare To Constant1/1, Compare To Constant2/1  "<HV_State>"
  Controls/1 -> Bus Selector1/1
  Unit Delay5/1 -> TriggerCompareTo/1
  Unit Delay1/1 -> TriggerCompareTo1/1
  Compare To Constant7/1 -> Unit Delay1/1
